simulink model "CANsimple"  (R2025b)
settings: Solver=VariableStepAuto  StartTime=0.0  StopTime=10.0  RelTol=1e-3
libraries: truetime x4
settings Model: Creator=ECC  LastModifiedBy=snorr
settings SolverCC: AlgebraicLoopSolver=TrustRegion
settings DataIOCC: ReturnWorkspaceOutputs=off
settings DebuggingCC: UnconnectedInputMsg=warning  UnconnectedOutputMsg=warning  UnconnectedLineMsg=warning  ArithmeticOperatorsInVariantConditions=warning
settings ModelReferenceCC: EnableRefExpFcnMdlSchedulingChecks=on
settings SFSimCC: SimUseLocalCustomCode=off  CustomCodeUndefinedFunction=UseInterfaceOnly
settings RTWCC: RTWUseLocalCustomCode=off  GPUComputeCapability=3.5

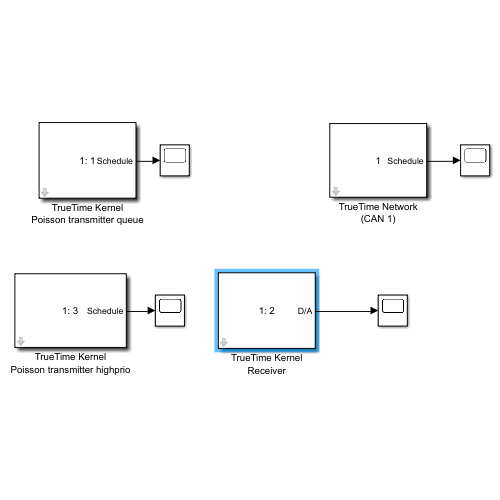
[thumbnail: Simulink's stored preview of the top-level diagram]
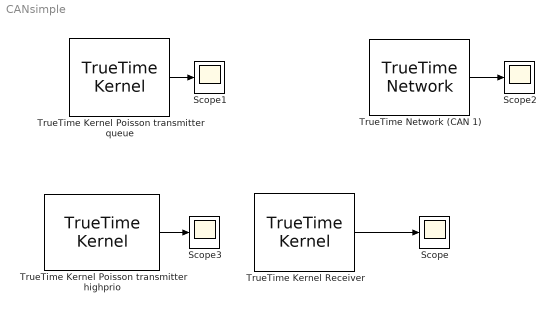
== system CANsimple ==
  Scope{,1..3} (4 alike) : Scope
      Scope settings: ActiveDisplayYMinimum=-1  ActiveDisplayYMaximum=1
      Scope1 settings: ActiveDisplayYMinimum=-1  ActiveDisplayYMaximum=1  DataLoggingVariableName=ScopeData2
      Scope2 settings: ActiveDisplayYMinimum=0.6875  ActiveDisplayYMaximum=3.8125
      Scope3 settings: ActiveDisplayYMinimum=-1  ActiveDisplayYMaximum=1  DataLoggingVariableName=ScopeData3
  TrueTime Kernel Poisson transmitter highprio : truetime/TrueTime Kernel  sfun=highprio_init  args=[]  ninputsoutputs=[0 0]  ntriggers=0  trigtype=falling  nwnodenbr=[1 3]  clockoffsetdrift=[0 0]  schedoutput=on  battery=off  poweroutput=off  label=1: 3
  TrueTime Kernel Poisson transmitter queue : truetime/TrueTime Kernel  Priority=1  sfun=transmitter_init  args=[]  ninputsoutputs=[0 0]  ntriggers=0  trigtype=rising  nwnodenbr=[1 1]  clockoffsetdrift=[0 0]  schedoutput=on  battery=off  poweroutput=off  label=1: 1
  TrueTime Kernel Receiver : truetime/TrueTime Kernel  Priority=1  sfun=receiver_init  args=[]  ninputsoutputs=[0 1]  ntriggers=0  trigtype=rising  nwnodenbr=[1 2]  clockoffsetdrift=[0 0]  schedoutput=off  battery=off  poweroutput=off  label=1: 2
  TrueTime Network (CAN 1) : truetime/TrueTime Network  Priority=1  nwtype=CSMA/AMP (CAN)  nwnbr=1  nnodes=3  rate=125000  minsize=29  lossprob=0  seed=0  bandwidths=[0.5 0.25 0.25]  slotsize=80  schedule=[1 2 1 3]  memsize=80000  buftype=Common buffer  overflow=Retransmit  dynSchedule=[]  miniSlotSize=40  NIT=0  QSortMode=FIFO  sync=0  irtSchedule=0  nrtLength=0  nodeGraph=0  scheduleoutput=on
  wires:
  TrueTime Network (CAN 1)/1 -> Scope2/1
  TrueTime Kernel Receiver/1 -> Scope/1
  TrueTime Kernel Poisson transmitter queue/1 -> Scope1/1
  TrueTime Kernel Poisson transmitter highprio/1 -> Scope3/1
